simulink library "rotationConversionLib"  (R2023b)
settings: Solver=VariableStepAuto  StartTime=0.0  StopTime=10.0  RelTol=1e-3
settings Model: Creator=kristopherriordan  LastModifiedBy=kristopherriordan

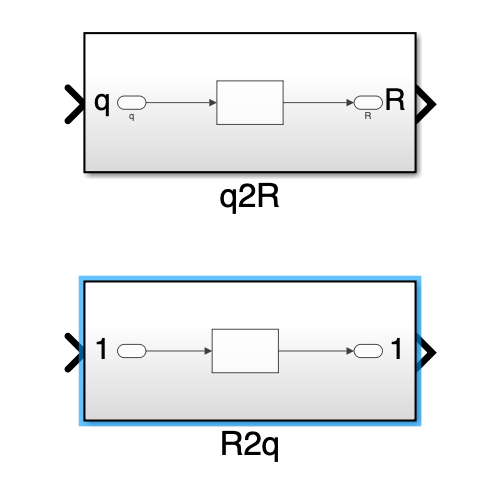
[thumbnail: Simulink's stored preview of the top-level diagram]
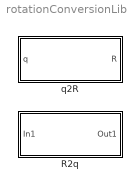
== system rotationConversionLib ==
  R2q : Subsystem
  q2R : Subsystem

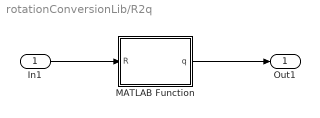
== system rotationConversionLib/R2q ==
  In1 : Inport
  MATLAB Function : MATLAB Function  TreatAsAtomicUnit=on
  Out1 : Outport
  wires:
  In1/1 -> MATLAB Function/1(R)
  MATLAB Function/1(q) -> Out1/1

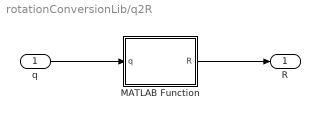
== system rotationConversionLib/q2R ==
  q : Inport
  MATLAB Function : MATLAB Function  TreatAsAtomicUnit=on
  R : Outport
  wires:
  q/1 -> MATLAB Function/1(q)
  MATLAB Function/1(R) -> R/1

== matlab function rotationConversionLib/q2R/MATLAB Function ==
  data: q input; R output
function R = q2R(q)

q0 = q(1);
q1 = q(2);
q2 = q(3);
q3 = q(4);

R = [q0^2 + q1^2 - q2^2 - q3^2, 2*q1*q2 + 2*q0 *q3, 2*(q1*q3 - q0*q2);
    2*(q1*q2 - q0*q3), q0^2 - q1^2 + q2^2 - q3^2, 2*(q2*q3 + q0*q1);
    2*(q1*q3 + q0*q2), 2*(q2*q3 - q0*q1), q0^2 - q1^2 - q2^2 + q3^2];

== matlab function rotationConversionLib/R2q/MATLAB Function ==
  data: R input; q output
function q = R2q(R)

q = zeros([4 1]);

if R(2,2) > -R(3,3) && R(1,1) > -R(2,2) && R(1,1) > -R(3,3)
    den = sqrt(1 + R(1,1) + R(2,2) + R(3,3));
    q = 0.5.*[den;
        (R(2,3) - R(3,2))/den;
        (R(3,1) - R(1,3))/den;
        (R(1,2) - R(2,1))/den];
elseif R(2,2) < -R(3,3) && R(1,1) > R(2,2) && R(1,1) > R(3,3)
    den = sqrt(1 + R(1,1) - R(2,2) - R(3,3));
    q = 0.5.*[(R(2,3) - R(3,2))/den;
        den;
        (R(1,2) + R(2,1))/den;
        (R(3,1) + R(1,3))/den];
elseif R(2,2) > R(3,3) && R(1,1) < R(2,2) && R(1,1) < -R(3,3)
    den = sqrt(1 - R(1,1) + R(2,2) - R(3,3));
    q = 0.5.*[(R(3,1) - R(1,3))/den;
        (R(1,2) + R(2,1))/den;
        den;
        (R(2,3) + R(3,2))/den];
elseif R(2,2) < R(3,3) && R(1,1) < -R(2,2) && R(1,1) < R(3,3)
    den = sqrt(1 - R(1,1) - R(2,2) + R(3,3));
    q = 0.5.*[(R(1,2) - R(2,1))/den;
        (R(3,1) + R(1,3))/den;
        (R(2,3) + R(3,2))/den;
        den];
end
